simulink model "USART_Rcv_And_Convert"  (R2013b)
settings: Solver=FixedStepDiscrete  StartTime=0.0  StopTime=10.0  FixedStep=0.5  RelTol=1e-3
undefined symbols (not defined in the file): PC10, PC11, uart4, usart3
libraries: USART_Lib x3
settings Model: Creator=reynaudp  LastModifiedBy=reynaudp
settings OptimizationCC: ExpressionDepthLimit=2147483647  OptimizeModelRefInitCode=on  LifeSpan=1
settings DebuggingCC: StateNameClashWarn=warning
settings HardwareCC: ProdLargestAtomicInteger=Integer  ProdLargestAtomicFloat=Float  ProdIntDivRoundTo=Zero  ProdEndianess=LittleEndian  ProdHWDeviceType=STMicroelectronics->STM32F4xx 32-bit Cortex-M4
settings RTWCC: SystemTargetFile=stm32F4xx.tlc  TemplateMakefile=stm32F4xx.tmf  Description=stm32F4xx (Embedded Target)  GenerateReport=on  ProcessScript=stm32F4xx_make_rtw_hook  IncludeHyperlinkInReport=on  LaunchReport=on
settings CodeAppCC: IgnoreCustomStorageClasses=off  CustomSymbolStrType=$N$R$M  InternalIdentifier=Classic
settings STFCustomTargetCC: ParMdlRefBuildCompliant=on  IncludeMdlTerminateFcn=off  CombineOutputUpdateFcns=on  ERTCustomFileBanners=on  SupportContinuousTime=off  SupportNonInlinedSFcns=off  SupportVariableSizeSignals=on  MATLABClassNameForMDSCustomization=Simulink.SoftwareTarget.ERTCustomization  GRTInterface=off  SystemTargetFile=stm32F4xx.tlc
settings ERTTargetCC: CodeReplacementLibrary=ANSI_C  CompOptLevelCompliant=off  ConcurrentExecutionCompliant=off  IncludeMdlTerminateFcn=off  ERTFirstTimeCompliant=off  SupportVariableSizeSignals=on  ModelStepFunctionPrototypeControlCompliant=off  CPPClassGenCompliant=off  InlinedParameterPlacement=NonHierarchical  ERTSrcFileBannerTemplate=sourceFileTemplate.cgt  ERTHdrFileBannerTemplate=sourceFileTemplate.cgt  ERTDataSrcFileTemplate=sourceFileTemplate.cgt  ERTDataHdrFileTemplate=sourceFileTemplate.cgt  ERTCustomFileTemplate=customRoutineProcess.tlc

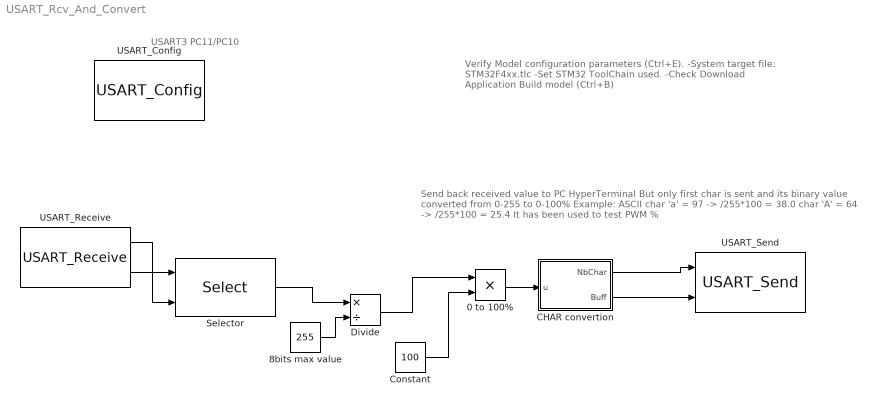
== system USART_Rcv_And_Convert ==
  note: Send back received value to PC
      | HyperTerminal
      | But only first char is sent and its binary value converted from 0-255 to 0-100%
      | Example: ASCII char 'a' =  97 -> /255*100 = 38.0
      |  char 'A' = 64 -> /255*100 = 25.4
      | It has been used to test PWM %
  note: USART3 PC11/PC10
  note: Verify Model configuration parameters (Ctrl+E).
      | 	-System target file: STM32F4xx.tlc
      | 	-Set STM32 ToolChain used.
      | 	-Check Download Application
      | Build model (Ctrl+B)
  0 to 100% : Product  RndMeth=Zero
  8bits max value : Constant  Value=255
  CHAR convertion : MATLAB Function  TreatAsAtomicUnit=on
  Constant : Constant  Value=100
  Divide : Product  Inputs=*/
  Selector : Selector  IndexMode=Zero-based  InputPortWidth=20  IndexOptions=Starting index (port)  Indices=[1 3]  OutputSizes=1
  USART_Config : USART_Lib/USART_Config  USART_CONFIG=USART3  USART_CONFIG_PIN=PC11/PC10 : (usart3 / uart4)  USART_SPEED=115200  USART_DATA=USART_WordLength_8b  USART_PARITY=USART_Parity_No  USART_STOP=USART_StopBits_1  USART_FLOW=off  USART_DEFAULT=off  It_rcv=on  It_send=on  Def_handler=on  Cust_handler=USART3_IRQHandler
  USART_Receive : USART_Lib/USART_Receive  USART_name=USART3  Buff_size=512  NbData_Size=20  Soft_it=off  Soft_num=0
  USART_Send : USART_Lib/USART_Send  USART_name=USART3  USART_buff=20
  wires:
  USART_Receive/2 -> Selector/1
  Selector/1 -> Divide/1
  8bits max value/1 -> Divide/2
  Divide/1 -> 0 to 100%/1
  USART_Receive/1 -> Selector/2
  CHAR convertion/1(NbChar) -> USART_Send/1
  CHAR convertion/2(Buff) -> USART_Send/2
  0 to 100%/1 -> CHAR convertion/1(u)
  Constant/1 -> 0 to 100%/2

== matlab function USART_Rcv_And_Convert/CHAR convertion ==
  data: u input; NbChar output uint16 size=1; Buff output uint8 size=[1 20]
function [NbChar, Buff] = convert(u)
%%Buff = uint32(0);
buffer = zeros(1,15,'uint8');
strLen = int32(0);
strLen = coder.ceval('sprintf',coder.wref(buffer),['%2.2f',0],u);
%tmp = buffer(1:strLen);
tmp = uint8('Volt');
y= [buffer(1:4), tmp, 13, 10, 0];
%%Buff = uint32(coder.ref(y));
Buff = [buffer(1:4), tmp, 13, 10, 0];
NbChar = uint16(size(y,2));
